simulink model "DevLib_ActrPrt"  (R2016b)
settings: configuration reference "CodeGenConfigSet" (kept outside this file)
values from neighbouring files (symbols this model uses):
  DebLib_nActrRls_C = Calibration.Parameter    [init_DevLib_ActrPrt.m]
  DevLib_tiActrPrt_C = Calibration.Parameter    [init_DevLib_ActrPrt.m]
undefined symbols (not defined in the file or in its folder): DevLib_ActrPrt_DT
settings Model: Creator=lenovo  LastModifiedBy=lenovo
settings ConfigSetRef: SourceLocation=Base Workspace

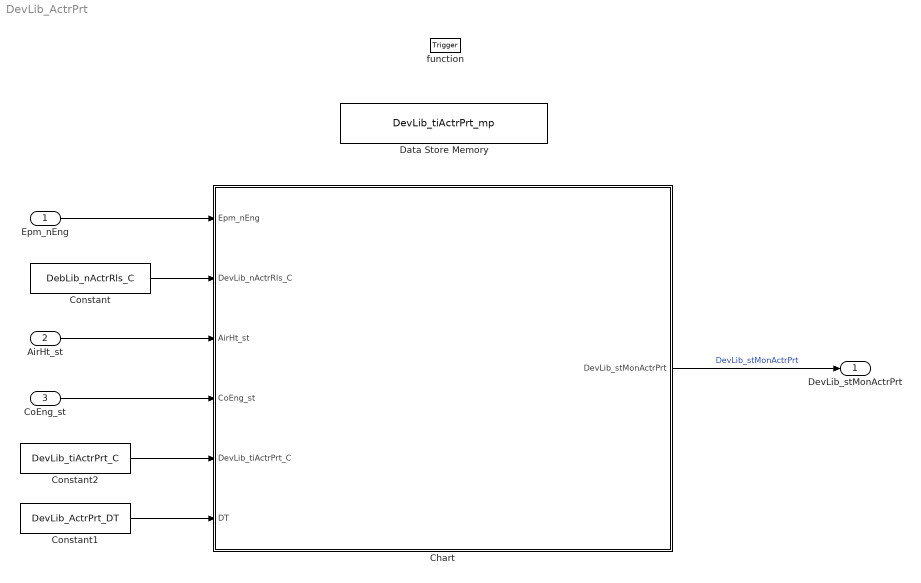
== system DevLib_ActrPrt ==
  Epm_nEng : Inport  Tag=rpm  Description=Engine speed  OutMin=0  OutMax=6000  OutDataTypeStr=EngSpeed_rpm
  AirHt_st : Inport  Description=status of AirHeater  Port=2  OutDataTypeStr=Enum: AirHtState_conv
  CoEng_st : Inport  Description=Engine coordinator state  Port=3  OutDataTypeStr=Enum: EngState_conv
  function : TriggerPort  TriggerType=function-call  VariantControl=Variant
  Chart : Stateflow chart
  Constant : Constant  Value=DebLib_nActrRls_C
  Constant1 : Constant  Value=DevLib_ActrPrt_DT  OutDataTypeStr=Inherit: Inherit via back propagation
  Constant2 : Constant  Value=DevLib_tiActrPrt_C
  Data Store Memory : DataStoreMemory  DataStoreName=DevLib_tiActrPrt_mp  ReadBeforeWriteMsg=warning  WriteAfterWriteMsg=warning  WriteAfterReadMsg=warning  ShowAdditionalParam=off  OutDataTypeStr=uint16
  DevLib_stMonActrPrt : Outport  Description=The current status of the actuator protection control  OutMin=0  OutMax=255  OutDataTypeStr=State_uint8
  wires:
  Chart/1(DevLib_stMonActrPrt) -> DevLib_stMonActrPrt/1  "DevLib_stMonActrPrt"
  Constant/1 -> Chart/2(DevLib_nActrRls_C)
  Constant2/1 -> Chart/5(DevLib_tiActrPrt_C)
  CoEng_st/1 -> Chart/4(CoEng_st)
  AirHt_st/1 -> Chart/3(AirHt_st)
  Epm_nEng/1 -> Chart/1(Epm_nEng)
  Constant1/1 -> Chart/6(DT)

== stateflow chart DevLib_ActrPrt/Chart ==
  state DEVLIB_ACTR_WAIT_STRT
    during:DevLib_stMonActrPrt = 0;
    DEVLIB_ACTR_WAIT_STRT -> (junction 32) [order 1]
    (junction 32) -> (junction 34) [order 1] : [(AirHt_st ~= AirHtState_conv.AIRHT_READING)&&...
        | (AirHt_st ~= AirHtState_conv.AIRHT_PREHTR)]
    (junction 34) -> (junction 38) [order 1] : [DevLib_tiActrPrt_mp < 65535]
    (junction 38) -> (junction 40) : {DevLib_tiActrPrt_mp = DevLib_tiActrPrt_mp + DT;}
    (junction 32) -> (junction 36) [order 2] : {DevLib_tiActrPrt_mp = 0;}
    (junction 34) -> (junction 40) [order 2]
    (junction 40) -> (junction 36)
  state DEVLIB_ACTR_PRT
    during:DevLib_stMonActrPrt = 64;
  state DEVLIB_ACTR_STRT_OPR
    during:DevLib_stMonActrPrt = 16;
    DEVLIB_ACTR_STRT_OPR -> (junction 50) [order 1]
    (junction 50) -> (junction 47) [order 1] : [Epm_nEng == 0]
    (junction 47) -> (junction 51) [order 1] : [DevLib_tiActrPrt_mp < 65535]
    (junction 51) -> (junction 53) : {DevLib_tiActrPrt_mp = DevLib_tiActrPrt_mp + DT;}
    (junction 50) -> (junction 44) [order 2] : {DevLib_tiActrPrt_mp = 0;}
    (junction 47) -> (junction 53) [order 2]
    (junction 53) -> (junction 44)
  state DEVLIB_ACTR_OPR
    during:DevLib_stMonActrPrt = 48;
  (default) -> DEVLIB_ACTR_WAIT_STRT : {DevLib_tiActrPrt_mp = uint16(0);}
  DEVLIB_ACTR_WAIT_STRT -> DEVLIB_ACTR_PRT [order 2] : [(AirHt_st ~= AirHtState_conv.AIRHT_READING)&&(AirHt_st ~= AirHtState_conv.AIRHT_PREHTR)&&...
      | (DevLib_tiActrPrt_mp >= DevLib_tiActrPrt_C)]
      | {DevLib_tiActrPrt_mp = 0;}
  DEVLIB_ACTR_WAIT_STRT -> DEVLIB_ACTR_STRT_OPR [order 1] : [Epm_nEng >= DevLib_nActrRls_C]
      | {DevLib_tiActrPrt_mp = 0;}
  DEVLIB_ACTR_PRT -> DEVLIB_ACTR_STRT_OPR : [Epm_nEng >= DevLib_nActrRls_C]
  DEVLIB_ACTR_STRT_OPR -> DEVLIB_ACTR_PRT [order 1] : [(DevLib_tiActrPrt_mp >= DevLib_tiActrPrt_C)&&...
      | (Epm_nEng == 0)]
  DEVLIB_ACTR_OPR -> DEVLIB_ACTR_PRT : [Epm_nEng == 0]
  DEVLIB_ACTR_STRT_OPR -> DEVLIB_ACTR_OPR [order 2] : [CoEng_st == EngState_conv.COENG_RUNNING]
  data: DevLib_stMonActrPrt output; Epm_nEng input; DevLib_nActrRls_C input; DevLib_tiActrPrt_mp data_store_memory; AirHt_st input; CoEng_st input; DevLib_tiActrPrt_C input; DT input
